simulink library "sf_bidder"  (Simulink 7.6)
settings: Solver=ode45  SolverMode=SingleTasking  StartTime=0.0  StopTime=10.0  RelTol=1e-3
settings Model: Creator=The MathWorks Inc.  CovMetricSettings=dcmtr  ExtModeAutoUpdateStatusClock=off

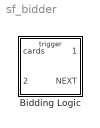
== system sf_bidder ==
  Bidding Logic : Stateflow chart  TreatAsAtomicUnit=on

== stateflow chart Bidding Logic ==
  state bid() [function]
    (default) -> (junction 18)
    (junction 18) -> (junction 19) : {
        | /* Open 1N */
        | aVarTruthTableCondition_1 = (point_count>=16&&point_count<=18);
        | }
    (junction 19) -> (junction 20) : {
        | /* Open 2N */
        | aVarTruthTableCondition_2 = (point_count>=20);
        | }
    (junction 20) -> (junction 21) : {
        | /* Open 2C */
        | aVarTruthTableCondition_3 = (total_points>=22);
        | }
    (junction 21) -> (junction 22) : {
        | /* Opening Count */
        | aVarTruthTableCondition_4 = (total_points>=13);
        | }
    (junction 22) -> (junction 23) : {
        | /* Premptable Count */
        | aVarTruthTableCondition_5 = (point_count>=6);
        | }
    (junction 23) -> (junction 24) : {
        | /* Bid Spades */
        | aVarTruthTableCondition_6 = (spade_count >= 5);
        | }
    (junction 24) -> (junction 25) : {
        | /* Bid Hearts */
        | aVarTruthTableCondition_7 = (heart_count >= 5);
        | }
    (junction 25) -> (junction 26) : {
        | /* Bid Diamonds */
        | aVarTruthTableCondition_8 = (diamond_count >= 4);
        | }
    (junction 26) -> (junction 27) : {
        | /* Preempt Spades */
        | aVarTruthTableCondition_9 = (spade_count >=6);
        | }
    (junction 27) -> (junction 28) : {
        | /* Preempt Hearts */
        | aVarTruthTableCondition_10 = (heart_count >=6);
        | }
    (junction 28) -> (junction 29) : {
        | /* Preempt Diamonds */
        | aVarTruthTableCondition_11 = (diamond_count >= 6);
        | }
    (junction 29) -> (junction 30) : {
        | /* Even Distribution */
        | aVarTruthTableCondition_12 = (distribution_count <= 1);
        | }
    (junction 30) -> (junction 31) [order 1] : [aVarTruthTableCondition_3 && !aVarTruthTableCondition_12]
    (junction 31) -> (junction 32) : {
        | /* Bid 2 */
        | bid_out += 2;
        | }
    (junction 32) -> (junction 33) : {
        | /* 'CLUBS':Bid Clubs */
        | bid_out += club_mask;
        | }
    (junction 30) -> (junction 34) [order 2]
    (junction 34) -> (junction 35) [order 1] : [aVarTruthTableCondition_2 && aVarTruthTableCondition_12]
    (junction 35) -> (junction 36) : {
        | /* Bid 2 */
        | bid_out += 2;
        | }
    (junction 36) -> (junction 37) : {
        | /* 'NO_TRUMP':Bid No Trump */
        | bid_out += no_trump_mask;
        | }
    (junction 34) -> (junction 38) [order 2]
    (junction 38) -> (junction 39) [order 1] : [aVarTruthTableCondition_1 && aVarTruthTableCondition_12]
    (junction 39) -> (junction 40) : {
        | /* Bid 1 */
        | bid_out += 1;
        | }
    (junction 40) -> (junction 41) : {
        | /* 'NO_TRUMP':Bid No Trump */
        | bid_out += no_trump_mask;
        | }
    (junction 38) -> (junction 42) [order 2]
    (junction 42) -> (junction 43) [order 1] : [aVarTruthTableCondition_4 && aVarTruthTableCondition_6]
    (junction 43) -> (junction 44) : {
        | /* Bid 1 */
        | bid_out += 1;
        | }
    (junction 44) -> (junction 45) : {
        | /* 'SPADES':Bid Spades */
        | bid_out += spade_mask;
        | }
    (junction 42) -> (junction 46) [order 2]
    (junction 46) -> (junction 47) [order 1] : [aVarTruthTableCondition_4 && aVarTruthTableCondition_7]
    (junction 47) -> (junction 48) : {
        | /* Bid 1 */
        | bid_out += 1;
        | }
    (junction 48) -> (junction 49) : {
        | /* 'HEARTS':Bid Hearts */
        | bid_out += heart_mask;
        | }
    (junction 46) -> (junction 50) [order 2]
    (junction 50) -> (junction 51) [order 1] : [aVarTruthTableCondition_4 && aVarTruthTableCondition_8]
    (junction 51) -> (junction 52) : {
        | /* Bid 1 */
        | bid_out += 1;
        | }
    (junction 52) -> (junction 53) : {
        | /* 'DIAMONDS':Bid Diamonds */
        | bid_out += diamond_mask;
        | }
    (junction 50) -> (junction 54) [order 2]
    (junction 54) -> (junction 55) [order 1] : [aVarTruthTableCondition_4]
    (junction 55) -> (junction 56) : {
        | /* Bid 1 */
        | bid_out += 1;
        | }
    (junction 56) -> (junction 57) : {
        | /* 'CLUBS':Bid Clubs */
        | bid_out += club_mask;
        | }
    (junction 54) -> (junction 58) [order 2]
    (junction 58) -> (junction 59) [order 1] : [aVarTruthTableCondition_5 && aVarTruthTableCondition_9]
    (junction 59) -> (junction 60) : {
        | /* Bid 2 */
        | bid_out += 2;
        | }
    (junction 60) -> (junction 61) : {
        | /* 'SPADES':Bid Spades */
        | bid_out += spade_mask;
        | }
    (junction 58) -> (junction 62) [order 2]
    (junction 62) -> (junction 63) [order 1] : [aVarTruthTableCondition_5 && aVarTruthTableCondition_10]
    (junction 63) -> (junction 64) : {
        | /* Bid 2 */
        | bid_out += 2;
        | }
    (junction 64) -> (junction 65) : {
        | /* 'HEARTS':Bid Hearts */
        | bid_out += heart_mask;
        | }
    (junction 62) -> (junction 66) [order 2]
    (junction 66) -> (junction 67) [order 1] : [aVarTruthTableCondition_5 && aVarTruthTableCondition_11]
    (junction 67) -> (junction 68) : {
        | /* Bid 2 */
        | bid_out += 2;
        | }
    (junction 68) -> (junction 69) : {
        | /* 'DIAMONDS':Bid Diamonds */
        | bid_out += diamond_mask;
        | }
    (junction 66) -> (junction 70) [order 2]
    (junction 70) -> (junction 71) : /* Default */
    (junction 71) -> (junction 72) : {
        | /* 'PASS':Pass */
        | bid_out = 0;
        | }
  state points = count_distribution(suit_count) [function]
    (junction 7) -> (junction 8) [order 1] : [suit_count < 3] {points = 3-suit_count;}
    (junction 7) -> (junction 6) [order 2] : {points = 0;}
    (default) -> (junction 7)
  (default) -> (junction 5) [order 1] : DEAL
      | {
      | loop = 0;
      | point_count = 0;
      | distribution_count = 0;
      | club_count = 0;
      | diamond_count = 0;
      | heart_count = 0;
      | spade_count = 0;
      | }
  (junction 5) -> (junction 11) [order 1] : [loop<13]
      | {
      | club_count += (cards[loop]&club_mask)>0;
      | diamond_count += (cards[loop]&diamond_mask)>0;
      | heart_count += (cards[loop]&heart_mask)>0;
      | spade_count += (cards[loop]&spade_mask)>0;
      | }
  (junction 5) -> (junction 9) [order 2]
  (default) -> (junction 10) [order 2] : BID
      | {bid_out = 0;}
  (junction 9) -> (junction 17) : {
      | distribution_count += count_distribution(club_count);
      | distribution_count += count_distribution(diamond_count);
      | distribution_count += count_distribution(heart_count);
      | distribution_count += count_distribution(spade_count);
      | total_points = distribution_count+point_count;
      | }
  (junction 13) -> (junction 5) : {loop++;}
  (junction 12) -> (junction 13)
  (junction 14) -> (junction 12)
  (junction 11) -> (junction 14) [order 1] : [cards[loop] & honor_mask]
      | {point_count+=cards[loop]&card_mask;}
  (junction 11) -> (junction 13) [order 2]
  (junction 10) -> (junction 16) [order 2] : {NEXT;}
  (junction 10) -> (junction 15) [order 1] : [bid_in == 0]
      | {bid();NEXT;}
  data: aVarTruthTableCondition_1 temporary boolean =0; aVarTruthTableCondition_2 temporary boolean =0; aVarTruthTableCondition_3 temporary boolean =0; aVarTruthTableCondition_4 temporary boolean =0; aVarTruthTableCondition_5 temporary boolean =0; aVarTruthTableCondition_6 temporary boolean =0; aVarTruthTableCondition_7 temporary boolean =0; aVarTruthTableCondition_8 temporary boolean =0; aVarTruthTableCondition_9 temporary boolean =0; aVarTruthTableCondition_10 temporary boolean =0; aVarTruthTableCondition_11 temporary boolean =0; aVarTruthTableCondition_12 temporary boolean =0; suit_count function_input double size=1; points function_output double size=1; club_mask constant uint8 size=1 =0x10; diamond_mask constant uint8 size=1 =0x20; heart_mask constant uint8 size=1 =0x40; spade_mask constant uint8 size=1 =0x80; honor_mask constant uint8 size=1 =0x08; point_count local uint8 size=1; club_count local uint8 size=1; diamond_count local uint8 size=1; heart_count local uint8 size=1; spade_count local uint8 size=1; distribution_count local uint8 size=1; total_points local uint8 size=1; loop local uint8 size=1; cards input uint8 size=13; card_mask constant uint8 size=1 =0x07; bid_in input uint8 size=1; bid_out output uint8 size=1; no_trump_mask constant uint8 size=1 =0x08
  data aVarTruthTableCondition_1 settings: description=Open 1N
  data aVarTruthTableCondition_2 settings: description=Open 2N
  data aVarTruthTableCondition_3 settings: description=Open 2C
  data aVarTruthTableCondition_4 settings: description=Opening Count
  data aVarTruthTableCondition_5 settings: description=Premptable Count
  data aVarTruthTableCondition_6 settings: description=Bid Spades
  data aVarTruthTableCondition_7 settings: description=Bid Hearts
  data aVarTruthTableCondition_8 settings: description=Bid Diamonds
  data aVarTruthTableCondition_9 settings: description=Preempt Spades
  data aVarTruthTableCondition_10 settings: description=Preempt Hearts
  data aVarTruthTableCondition_11 settings: description=Preempt Diamonds
  data aVarTruthTableCondition_12 settings: description=Even Distribution
  events: DEAL input EITHER_EDGE_EVENT; BID input EITHER_EDGE_EVENT; NEXT output EITHER_EDGE_EVENT
